simulink model "Buzzer_harness"  (Simulink 7.7)
settings: Solver=FixedStepDiscrete  SolverMode=SingleTasking  StartTime=0.0  StopTime=100  FixedStep=.01  RelTol=1e-3
PostLoadFcn:
  | cd '..';
  | PostLoadFcn;
  | cd 'harness';
undefined symbols (not defined in the file): ACTIVE, BEEP_NONE, CONTINUOUS_BEEP, DOUBLE_SHORT_BEEP, INACTIVE, NO_BEEP, sigbuilder_block, SINGLE_LONG_BEEP, SINGLE_MEDIUM_BEEP, SINGLE_SHORT_BEEP, srate, SYS_NORMAL, TRIPLE_SHORT_BEEP
settings Model: Creator=smindema  LastModifiedBy=aliebel  CovMetricSettings=dcmw  CovHTMLOptions=-aTS=1 -bRG=1 -bTC=1 -hTR=0 -nFC=0 -scm=1 -bcm=1 -xEv=0  covSaveCumulativeToWorkspaceVar=off  CovSaveSingleToWorkspaceVar=off
settings MATStruct: SampleTime=0.01  Offset=0  Priority=[1.0]
settings DataIOCC: LimitDataPoints=off  SaveOutput=off  SaveTime=off
settings OptimizationCC: BlockReduction=off  InlineParams=on  ExpressionFolding=off  StateBitsets=on  DataBitsets=on  UseTempVars=on  InitFltsAndDblsToZero=on  NoFixptDivByZeroProtection=on  EfficientFloat2IntCast=on  OptimizeModelRefInitCode=on
settings DebuggingCC: SaveWithParameterizedLinksMsg=none  MultiTaskDSMMsg=warning  MultiTaskCondExecSysMsg=none  IntegerOverflowMsg=none  ModelReferenceCSMismatchMessage=warning
settings HardwareCC: ProdBitPerInt=16  ProdBitPerPointer=16  ProdIntDivRoundTo=Floor  ProdEndianess=BigEndian  ProdWordSize=16  ProdHWDeviceType=Motorola HC12
settings ModelReferenceCC: ModelReferenceNumInstancesAllowed=Single
settings RTWCC: SystemTargetFile=ert.tlc  GenCodeOnly=on  TemplateMakefile=ert_default_tmf  Description=Real-Time Workshop Embedded Coder (no auto configuration)  GenerateReport=on  RetainRTWFile=on  ProcessScript=ert_make_rtw_hook  IncludeHyperlinkInReport=on  LaunchReport=on  IncludeERTFirstTime=on
settings RTWCC: CustomHeaderCode=|
  | #include "cpp_req_defines.h"
  | #include "hw_fin.h"
  | #include "cdata.h"
settings CodeAppCC: IgnoreCustomStorageClasses=off  DefineNamingRule=UpperCase
settings ERTTargetCC: TargetFcnLib=ansi_tfl_tmw.mat  FunctionExecutionProfile=off  MultiwordLength=2048  GenerateSampleERTMain=on  IncludeMdlTerminateFcn=off  SupportAbsoluteTime=off  SupportNonFinite=off  SupportComplex=off  PurelyIntegerCode=on  ERTCustomFileTemplate=gen_rtw_req_defines_h.tlc  GlobalDataDefinition=InSeparateSourceFile  GlobalDataReference=InSeparateHeaderFile  ConvertIfToSwitch=off

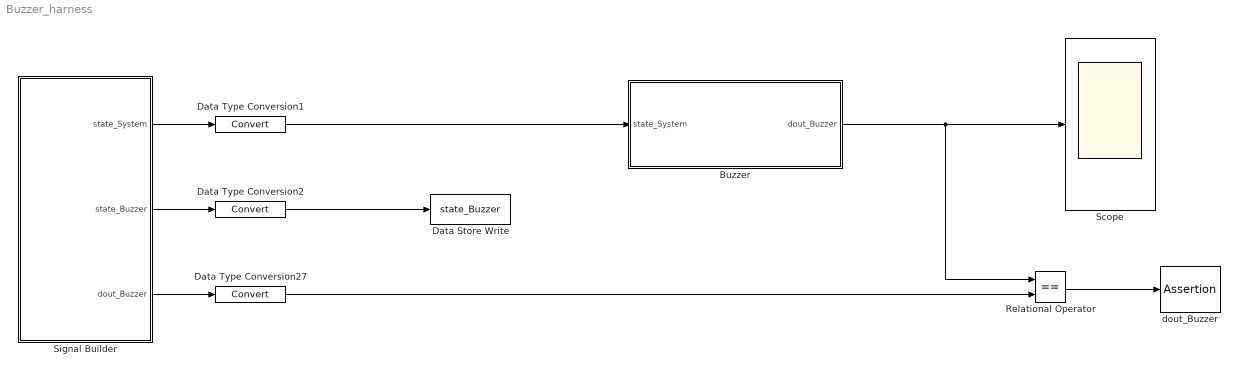
== system Buzzer_harness ==
  Buzzer : Subsystem  TreatAsAtomicUnit=on  SystemSampleTime=srate  RTWFileName=mod_Outputs
      settings: RTWSystemCode=Function  RTWFileNameOpts=User specified
  Data Store Write : DataStoreWrite  DataStoreName=state_Buzzer
  Data Type Conversion1 : DataTypeConversion
  Data Type Conversion2 : DataTypeConversion
  Data Type Conversion27 : DataTypeConversion
  Relational Operator : RelationalOperator  Operator===  OutDataTypeStr=boolean
  Scope : Scope
      settings: TimeRange=100  YMin=0  YMax=6  DataFormat=Array
  Signal Builder : Subsystem  Tag=STV Subsys  LoadFcn=sigbuilder_block('load',[381 256.5 911.25 362.25 ]);  StartFcn=sigbuilder_block('start');  StopFcn=sigbuilder_block('stop');  ClipboardFcn=sigbuilder_block('clipboard');  mask(Sigbuilder block){}
      mask help: Create and generate interchangeable groups of signals whose waveforms are piecewise linear.
      mask init:
      | if ~strcmp(get_param(bdroot(gcbh),'SimulationStatus'),'stopped') tuvar = sigbuilder_block('maskInit'); end
      settings: CopyFcn=sigbuilder_block('copy');  DeleteFcn=sigbuilder_block('delete');  ModelCloseFcn=sigbuilder_block('modelClose');  PreSaveFcn=sigbuilder_block('preSave');  NameChangeFcn=sigbuilder_block('namechange');  OpenFcn=sigbuilder_block('open',[118.5 149.25 911.25 362.25 ]);  CloseFcn=sigbuilder_block('close');
      mask Display: plot(0, 0, 100, 100,[2, 2, 32, 32, 2], [68, 8, 8, 68, 68],[32, 2], [38, 38], [32, 19, 2],[53, 60, 44], [32, 17, 17, 2],[16, 16, 31, 31]);txt = getActiveGroup(gcbh);text(2, 100, txt,'verticalAlignment', 'top');
  dout_Buzzer : Assertion  Enabled=off
  wires:
  Data Type Conversion27/1 -> Relational Operator/2
  Data Type Conversion2/1 -> Data Store Write/1
  Signal Builder/1(state_System) -> Data Type Conversion1/1
  Signal Builder/2(state_Buzzer) -> Data Type Conversion2/1
  Signal Builder/3(dout_Buzzer) -> Data Type Conversion27/1
  Buzzer/1(dout_Buzzer) -> Scope/1, Relational Operator/1
  Data Type Conversion1/1 -> Buzzer/1(state_System)
  Relational Operator/1 -> dout_Buzzer/1

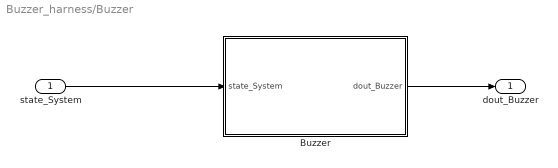
== system Buzzer_harness/Buzzer ==
  state_System : Inport  OutDataTypeStr=uint8
  Buzzer : Stateflow chart  RTWFileName=mod_Diagnostics
      settings: RTWSystemCode=Function  RTWFileNameOpts=User specified
  dout_Buzzer : Outport
  wires:
  Buzzer/1(dout_Buzzer) -> dout_Buzzer/1
  state_System/1 -> Buzzer/1(state_System)

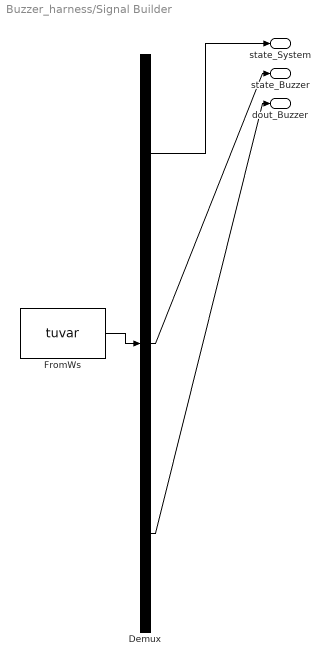
== system Buzzer_harness/Signal Builder ==
  Demux : Demux  Tag=STV Demux  Outputs=3
  FromWs : FromWorkspace  Tag=STV FromWs  VariableName=tuvar  SampleTime=0  SigBuilderData=DataTag0  VnvData=DataTag1
      SigBuilderData=|
      | common.afterFinalStr = 'Extrapolate'
      | common.sampleTime = 0
      | dataSet(1).timeRange = [0 100]
      | dataSet(1).name = 'Continuous'
      | dataSet(2).timeRange = [0 100]
      | dataSet(2).name = 'Multiple_Short'
      | dataSet(3).timeRange = [0 100]
      | dataSet(3).name = 'Medium_Long'
      | sbobj.Groups(1).Name = 'Continuous'
      | sbobj.Groups(1).Signals(1).Name = 'state_System'
      | sbobj.Groups(1).Signals(1).XData = [0 9 9 100]
      | sbobj.Groups(1).Signals(1).YData = [0 0 1 1]
      | sbobj.Groups(1).Signals(2).Name = 'state_Buzzer'
      | sbobj.Groups(1).Signals(2).XData = [0 1.22 1.22 2.27 2.27 3.32 3.32 12.55 12.55 16.43 16.43 100]
      | sbobj.Groups(1).Signals(2).YData = [255 255 0 0 1 1 255 255 1 1 255 255]
      | sbobj.Groups(1).Signals(3).Name = 'dout_Buzzer'
      | sbobj.Groups(1).Signals(3).XData = [0 100]
      | sbobj.Groups(1).Signals(3).YData = [0 0]
      | sbobj.Groups(1).TimeRange = [0 100]
      | sbobj.Groups(2).Name = 'Multiple_Short'
      | sbobj.Groups(2).Signals(1).Name = 'state_System'
      | sbobj.Groups(2).Signals(1).XData = [0 100]
      | sbobj.Groups(2).Signals(1).YData = [1 1]
      | sbobj.Groups(2).Signals(2).Name = 'state_Buzzer'
      | sbobj.Groups(2).Signals(2).XData = [0 5 5 5.1 5.1 10 10 10.4 10.4 15 15 15.7 15.7 100]
      | sbobj.Groups(2).Signals(2).YData = [0 0 16 16 0 0 32 32 0 0 48 48 0 0]
      | sbobj.Groups(2).Signals(3).Name = 'dout_Buzzer'
      | sbobj.Groups(2).Signals(3).XData = [0 100]
      | sbobj.Groups(2).Signals(3).YData = [0 0]
      | sbobj.Groups(2).TimeRange = [0 100]
      | sbobj.Groups(3).Name = 'Medium_Long'
      | sbobj.Groups(3).Signals(1).Name = 'state_System'
      | sbobj.Groups(3).Signals(1).XData = [0 52 52 54 54 55.2 55.2 56 56 61 61 62 62 70 70 72.21 72.21 100]
      | sbobj.Groups(3).Signals(1).YData = [1 1 0 0 1 1 0 0 1 1 0 0 1 1 0 0 1 1]
      | sbobj.Groups(3).Signals(2).Name = 'state_Buzzer'
      | sbobj.Groups(3).Signals(2).XData = [0 5 5 6.01 6.01 10 10 10.5 10.5 11.3 11.3 15 15 15.4 15.4 16.3 16.3 20 20 35 35 37 37 37.01 37.01 45 45 45.1 45.1 50 50 52.01 52.01 55 55 55.21 55.21 60 60 60.6 60.6 60.66 60.66 65 65 70.01 70.01 100]
      | sbobj.Groups(3).Signals(2).YData = [0 0 19 19 0 0 19 19 48 48 0 0 19 19 48 48 0 0 31 31 0 0 15 15 0 0 31 31 0 0 31 31 0 0 48 48 0 0 19 19 48 48 0 0 1 1 0 0]
      | sbobj.Groups(3).Signals(3).Name = 'dout_Buzzer'
      | sbobj.Groups(3).Signals(3).XData = [0 100]
      | sbobj.Groups(3).Signals(3).YData = [0 0]
      | sbobj.Groups(3).TimeRange = [0 100]
  state_System : Outport  Tag=STV Outport
  state_Buzzer : Outport  Tag=STV Outport  Port=2
  dout_Buzzer : Outport  Tag=STV Outport  Port=3
  wires:
  Demux/1 -> state_System/1
  FromWs/1 -> Demux/1
  Demux/2 -> state_Buzzer/1
  Demux/3 -> dout_Buzzer/1

== stateflow chart Buzzer/Buzzer ==
  settings: updateMethod=DISCRETE  sampleTime=srate
  state No_Beep
    en:
    dout_Buzzer = INACTIVE;
    state_Buzzer = NO_BEEP;
    Beeps = 0;
  state Beep
    state Multiple_Off
      en:
      dout_Buzzer = INACTIVE;
    state One_Beep_Medium
      en:
      dout_Buzzer = ACTIVE;
      on after(ONE_SECOND, tick):
      Beeps = 0;
    state Multiple_On
      en:
      dout_Buzzer = ACTIVE;
    state On
      en:
      dout_Buzzer = ACTIVE;
    state Brief_Off
      en:
      dout_Buzzer = INACTIVE;
    state One_Beep_Long
      en:
      dout_Buzzer = ACTIVE;
      on after(FIFTEEN_SECONDS, tick):
      Beeps = 0;
    Multiple_Off -> Multiple_On : [after(20,tick)]
    (junction 14) -> Multiple_On [order 1] : [state_Buzzer == TRIPLE_SHORT_BEEP]
        | {Beeps = 3;}
    One_Beep_Medium -> Brief_Off : [state_Buzzer == TRIPLE_SHORT_BEEP...
        | && after(50, tick)]
        | {Beeps = 3;}
    (junction 15) -> One_Beep_Medium [order 1] : [state_Buzzer == SINGLE_MEDIUM_BEEP]
        | {Beeps = 1;}
    (junction 14) -> (junction 15) [order 2]
    Brief_Off -> Multiple_On : [after(10,tick)]
    (junction 13) -> Multiple_On [order 1] : [state_Buzzer == SINGLE_SHORT_BEEP]
        | {Beeps = 1;}
    (junction 11) -> Multiple_On [order 1] : [state_Buzzer == DOUBLE_SHORT_BEEP]
        | {Beeps = 2;}
    Multiple_On -> Multiple_Off : [after(10,tick)]
        | {Beeps--;}
    (junction 12) -> On [order 1] : [state_Buzzer == CONTINUOUS_BEEP]
        | {Beeps = 1;}
    (junction 12) -> (junction 13) [order 2]
    (junction 13) -> (junction 11) [order 2]
    (junction 11) -> (junction 14) [order 2]
    (junction 16) -> One_Beep_Long [order 1] : [state_Buzzer == SINGLE_LONG_BEEP]
        | {Beeps = 1;}
    (junction 15) -> (junction 16) [order 2]
  No_Beep -> (junction 12) : [state_Buzzer != BEEP_NONE...
      | && state_Buzzer != NO_BEEP...
      | && state_System == SYS_NORMAL]
  Beep -> No_Beep : [state_Buzzer == NO_BEEP...
      | || !Beeps...
      | || state_System != SYS_NORMAL]
  (junction 16) -> No_Beep [order 2]
  (default) -> No_Beep
  data: dout_Buzzer output boolean; Beeps local uint8; NO_BEEP parameter uint8; SINGLE_MEDIUM_BEEP parameter uint8; TRIPLE_SHORT_BEEP parameter uint8; DOUBLE_SHORT_BEEP parameter uint8; SINGLE_SHORT_BEEP parameter uint8; ONE_SECOND constant uint16 =99; CONTINUOUS_BEEP parameter uint8; ACTIVE parameter uint8; INACTIVE parameter uint8; state_Buzzer data_store_memory double; state_System input uint8; SYS_NORMAL parameter uint8; SINGLE_LONG_BEEP parameter uint8; FIFTEEN_SECONDS constant uint16 =1499; BEEP_NONE parameter uint8
